simulink model "w3_warplab_buffers"  (Simulink 7.7)
settings: Solver=VariableStepDiscrete  SolverMode=SingleTasking  StartTime=0.0  StopTime=200000  RelTol=1e-3
InitFcn:
  | w3_warplab_buffers_init
StartFcn:
  | w3_warplab_buffers_init
values from neighbouring files (symbols this model uses):
  NumSamps_Rx_IQ = 2^15    (= 32768)    [w3_warplab_buffers_init.m]
  NumSamps_Rx_RSSI = 2^13    (= 8192)    [w3_warplab_buffers_init.m]
  NumSamps_Tx_IQ = 2^15    (= 32768)    [w3_warplab_buffers_init.m]
undefined symbols (not defined in the file or in its folder): gcbh, xlBlockLoadCallback, xlGetNormalizedPeriod
libraries: xbsIndex_r4 x1266, xbsEDKLib_r4 x1
(part 6 of 9)

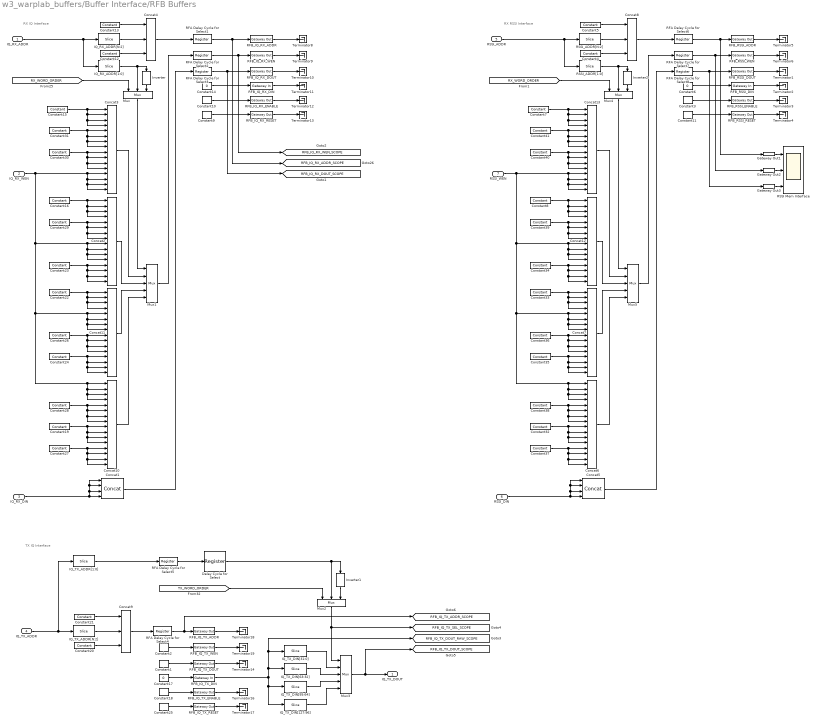
== system w3_warplab_buffers/Buffer Interface/RFB Buffers ==
  note: RX IQ Interface
  note: TX IQ Interface
  note: RX RSSI Interface
  IQ_RX_ADDR : Inport
  IQ_RX_WEN : Inport  Port=2
  IQ_RX_DIN : Inport  Port=3
  IQ_TX_ADDR : Inport  Port=4
  RSSI_ADDR : Inport  Port=5
  RSSI_DIN : Inport  Port=6
  RSSI_WEN : Inport  Port=7
  Concat1 : xbsIndex_r4/Concat  num_inputs=4  dbl_ovrd=off  block_type=concat
  Concat{2..3,6..7,10..13} (8 alike) : xbsIndex_r4/Concat  num_inputs=16  dbl_ovrd=off  block_type=concat
  Concat4 : xbsIndex_r4/Concat  num_inputs=3  dbl_ovrd=off  block_type=concat
  Concat5 : xbsIndex_r4/Concat  num_inputs=4  dbl_ovrd=off  block_type=concat
  Concat8 : xbsIndex_r4/Concat  num_inputs=3  dbl_ovrd=off  block_type=concat
  Concat9 : xbsIndex_r4/Concat  num_inputs=3  dbl_ovrd=off  block_type=concat
  Constant1 : xbsIndex_r4/Constant  const=0  gui_display_data_type=Fixed-point  arith_type=Unsigned  n_bits=128  bin_pt=0  preci_type=Single  exp_width=8  frac_width=24  explicit_period=off  period=1  equ=P=C  opselect=C  inp2=PCIN>>17  opr=+  inp1=P  carry=CIN  dbl_ovrd=off  block_type=constant
      settings: block_version=10.1.2
  Constant10 : xbsIndex_r4/Constant  const=1  gui_display_data_type=Boolean  arith_type=Boolean  n_bits=32  bin_pt=0  preci_type=Single  exp_width=8  frac_width=24  explicit_period=off  period=1  equ=P=C  opselect=C  inp2=PCIN>>17  opr=+  inp1=P  carry=CIN  dbl_ovrd=off  block_type=constant
      settings: block_version=10.1.2
  Constant11 : xbsIndex_r4/Constant  const=0  gui_display_data_type=Boolean  arith_type=Boolean  n_bits=32  bin_pt=0  preci_type=Single  exp_width=8  frac_width=24  explicit_period=off  period=1  equ=P=C  opselect=C  inp2=PCIN>>17  opr=+  inp1=P  carry=CIN  dbl_ovrd=off  block_type=constant
      settings: block_version=10.1.2
  Constant12 : xbsIndex_r4/Constant  const=0  gui_display_data_type=Fixed-point  arith_type=Unsigned  n_bits=4  bin_pt=0  preci_type=Single  exp_width=8  frac_width=24  explicit_period=off  period=1  equ=P=C  opselect=C  inp2=PCIN>>17  opr=+  inp1=P  carry=CIN  dbl_ovrd=off  block_type=constant
  Constant13 : xbsIndex_r4/Constant  const=0  gui_display_data_type=Fixed-point  arith_type=Unsigned  n_bits=30 - ceil(log2(NumSamps_Rx_IQ))  bin_pt=0  preci_type=Single  exp_width=8  frac_width=24  explicit_period=off  period=1  equ=P=C  opselect=C  inp2=PCIN>>17  opr=+  inp1=P  carry=CIN  dbl_ovrd=off  block_type=constant
  Constant14 : Constant  Value=0
  Constant{7..8,15..16,19,22..24,26..41} (24 alike) : xbsIndex_r4/Constant  const=0  gui_display_data_type=Boolean  arith_type=Boolean  n_bits=1  bin_pt=0  preci_type=Single  exp_width=8  frac_width=24  explicit_period=off  period=1  equ=P=C  opselect=C  inp2=PCIN>>17  opr=+  inp1=P  carry=CIN  dbl_ovrd=off  block_type=constant
  Constant17 : Constant  Value=0
  Constant18 : xbsIndex_r4/Constant  const=1  gui_display_data_type=Boolean  arith_type=Boolean  n_bits=32  bin_pt=0  preci_type=Single  exp_width=8  frac_width=24  explicit_period=off  period=1  equ=P=C  opselect=C  inp2=PCIN>>17  opr=+  inp1=P  carry=CIN  dbl_ovrd=off  block_type=constant
      settings: block_version=10.1.2
  Constant2 : xbsIndex_r4/Constant  const=0  gui_display_data_type=Fixed-point  arith_type=Unsigned  n_bits=16  bin_pt=0  preci_type=Single  exp_width=8  frac_width=24  explicit_period=off  period=1  equ=P=C  opselect=C  inp2=PCIN>>17  opr=+  inp1=P  carry=CIN  dbl_ovrd=off  block_type=constant
      settings: block_version=10.1.2
  Constant20 : xbsIndex_r4/Constant  const=0  gui_display_data_type=Fixed-point  arith_type=Unsigned  n_bits=4  bin_pt=0  preci_type=Single  exp_width=8  frac_width=24  explicit_period=off  period=1  equ=P=C  opselect=C  inp2=PCIN>>17  opr=+  inp1=P  carry=CIN  dbl_ovrd=off  block_type=constant
  Constant21 : xbsIndex_r4/Constant  const=0  gui_display_data_type=Fixed-point  arith_type=Unsigned  n_bits=30 - ceil(log2(NumSamps_Tx_IQ))  bin_pt=0  preci_type=Single  exp_width=8  frac_width=24  explicit_period=off  period=1  equ=P=C  opselect=C  inp2=PCIN>>17  opr=+  inp1=P  carry=CIN  dbl_ovrd=off  block_type=constant
  Constant25 : xbsIndex_r4/Constant  const=0  gui_display_data_type=Boolean  arith_type=Boolean  n_bits=32  bin_pt=0  preci_type=Single  exp_width=8  frac_width=24  explicit_period=off  period=1  equ=P=C  opselect=C  inp2=PCIN>>17  opr=+  inp1=P  carry=CIN  dbl_ovrd=off  block_type=constant
      settings: block_version=10.1.2
  Constant3 : xbsIndex_r4/Constant  const=1  gui_display_data_type=Boolean  arith_type=Boolean  n_bits=32  bin_pt=0  preci_type=Single  exp_width=8  frac_width=24  explicit_period=off  period=1  equ=P=C  opselect=C  inp2=PCIN>>17  opr=+  inp1=P  carry=CIN  dbl_ovrd=off  block_type=constant
      settings: block_version=10.1.2
  Constant4 : xbsIndex_r4/Constant  const=0  gui_display_data_type=Fixed-point  arith_type=Unsigned  n_bits=4  bin_pt=0  preci_type=Single  exp_width=8  frac_width=24  explicit_period=off  period=1  equ=P=C  opselect=C  inp2=PCIN>>17  opr=+  inp1=P  carry=CIN  dbl_ovrd=off  block_type=constant
  Constant5 : xbsIndex_r4/Constant  const=0  gui_display_data_type=Fixed-point  arith_type=Unsigned  n_bits=31 - ceil(log2(NumSamps_Rx_RSSI))  bin_pt=0  preci_type=Single  exp_width=8  frac_width=24  explicit_period=off  period=1  equ=P=C  opselect=C  inp2=PCIN>>17  opr=+  inp1=P  carry=CIN  dbl_ovrd=off  block_type=constant
  Constant6 : Constant  Value=0
  Constant9 : xbsIndex_r4/Constant  const=0  gui_display_data_type=Boolean  arith_type=Boolean  n_bits=32  bin_pt=0  preci_type=Single  exp_width=8  frac_width=24  explicit_period=off  period=1  equ=P=C  opselect=C  inp2=PCIN>>17  opr=+  inp1=P  carry=CIN  dbl_ovrd=off  block_type=constant
      settings: block_version=10.1.2
  Delay Cycle for Select : xbsIndex_r4/Register  init=0  rst=off  en=off  dbl_ovrd=off  block_type=register
  Gateway Out1 : xbsIndex_r4/Gateway Out  inherit_from_input=off  hdl_port=off  timing_constraint=None  locs_specified=off  LOCs={}  UseAsDAC=off  DACChannel='1'  block_type=gatewayout
      settings: infoedit="Gateway out block.  Converts Xilinx fixed point inputs into ouputs of type Simulink integer, double, or fixed point.<P><P>Hardware notes:  In hardware these blocks become top level output ports or are discarded, depending on how they are configured."  block_version=10.1.2
  Gateway Out2 : xbsIndex_r4/Gateway Out  inherit_from_input=off  hdl_port=off  timing_constraint=None  locs_specified=off  LOCs={}  UseAsDAC=off  DACChannel='1'  block_type=gatewayout
      settings: infoedit="Gateway out block.  Converts Xilinx fixed point inputs into ouputs of type Simulink integer, double, or fixed point.<P><P>Hardware notes:  In hardware these blocks become top level output ports or are discarded, depending on how they are configured."  block_version=10.1.2
  Gateway Out3 : xbsIndex_r4/Gateway Out  inherit_from_input=off  hdl_port=off  timing_constraint=None  locs_specified=off  LOCs={}  UseAsDAC=off  DACChannel='1'  block_type=gatewayout
      settings: infoedit="Gateway out block.  Converts Xilinx fixed point inputs into ouputs of type Simulink integer, double, or fixed point.<P><P>Hardware notes:  In hardware these blocks become top level output ports or are discarded, depending on how they are configured."  block_version=10.1.2
  IQ_RX_ADDR[1:0] : xbsIndex_r4/Slice  nbits=2  boolean_output=off  mode=Lower Bit Location + Width  bit1=0  base1=MSB of Input  bit0=0  base0=LSB of Input  dbl_ovrd=off  block_type=slice
  IQ_RX_ADDR[N:2] : xbsIndex_r4/Slice  nbits=ceil(log2(NumSamps_Rx_IQ)) - 2  boolean_output=off  mode=Lower Bit Location + Width  bit1=0  base1=MSB of Input  bit0=2  base0=LSB of Input  dbl_ovrd=off  block_type=slice
  IQ_TX_ADDR[1:0] : xbsIndex_r4/Slice  nbits=2  boolean_output=off  mode=Lower Bit Location + Width  bit1=0  base1=MSB of Input  bit0=0  base0=LSB of Input  dbl_ovrd=off  block_type=slice
  IQ_TX_ADDR[N:2] : xbsIndex_r4/Slice  nbits=ceil(log2(NumSamps_Tx_IQ)) - 2  boolean_output=off  mode=Lower Bit Location + Width  bit1=0  base1=MSB of Input  bit0=2  base0=LSB of Input  dbl_ovrd=off  block_type=slice
  IQ_TX_DIN[127:96] : xbsIndex_r4/Slice  nbits=32  boolean_output=off  mode=Lower Bit Location + Width  bit1=0  base1=MSB of Input  bit0=96  base0=LSB of Input  dbl_ovrd=off  block_type=slice
  IQ_TX_DIN[31:0] : xbsIndex_r4/Slice  nbits=32  boolean_output=off  mode=Lower Bit Location + Width  bit1=0  base1=MSB of Input  bit0=0  base0=LSB of Input  dbl_ovrd=off  block_type=slice
  IQ_TX_DIN[63:32] : xbsIndex_r4/Slice  nbits=32  boolean_output=off  mode=Lower Bit Location + Width  bit1=0  base1=MSB of Input  bit0=32  base0=LSB of Input  dbl_ovrd=off  block_type=slice
  IQ_TX_DIN[95:64] : xbsIndex_r4/Slice  nbits=32  boolean_output=off  mode=Lower Bit Location + Width  bit1=0  base1=MSB of Input  bit0=64  base0=LSB of Input  dbl_ovrd=off  block_type=slice
  Inverter : xbsIndex_r4/Inverter  en=off  latency=0  dbl_ovrd=off  block_type=inv
  Inverter1 : xbsIndex_r4/Inverter  en=off  latency=0  dbl_ovrd=off  block_type=inv
  Inverter2 : xbsIndex_r4/Inverter  en=off  latency=0  dbl_ovrd=off  block_type=inv
  Mux : xbsIndex_r4/Mux  inputs=2  en=off  latency=0  precision=Full  arith_type=Unsigned  n_bits=16  bin_pt=14  quantization=Truncate  overflow=Wrap  dbl_ovrd=off  block_type=mux
  Mux1 : xbsIndex_r4/Mux  inputs=4  en=off  latency=0  precision=Full  arith_type=Unsigned  n_bits=16  bin_pt=14  quantization=Truncate  overflow=Wrap  dbl_ovrd=off  block_type=mux
  Mux2 : xbsIndex_r4/Mux  inputs=2  en=off  latency=0  precision=Full  arith_type=Unsigned  n_bits=16  bin_pt=14  quantization=Truncate  overflow=Wrap  dbl_ovrd=off  block_type=mux
  Mux3 : xbsIndex_r4/Mux  inputs=4  en=off  latency=0  precision=Full  arith_type=Unsigned  n_bits=16  bin_pt=14  quantization=Truncate  overflow=Wrap  dbl_ovrd=off  block_type=mux
  Mux4 : xbsIndex_r4/Mux  inputs=2  en=off  latency=0  precision=Full  arith_type=Unsigned  n_bits=16  bin_pt=14  quantization=Truncate  overflow=Wrap  dbl_ovrd=off  block_type=mux
  Mux5 : xbsIndex_r4/Mux  inputs=4  en=off  latency=0  precision=Full  arith_type=Unsigned  n_bits=16  bin_pt=14  quantization=Truncate  overflow=Wrap  dbl_ovrd=off  block_type=mux
  RFA Delay Cycle for Select{1..8} (8 alike) : xbsIndex_r4/Register  init=0  rst=off  en=off  dbl_ovrd=off  block_type=register
  RFB_IQ_RX_ADDR : xbsIndex_r4/Gateway Out  inherit_from_input=off  hdl_port=on  timing_constraint=None  locs_specified=off  LOCs={}  UseAsDAC=off  DACChannel='1'  block_type=gatewayout
  RFB_IQ_RX_DIN : xbsIndex_r4/Gateway In  gui_display_data_type=Fixed-point  arith_type=Unsigned  n_bits=128  bin_pt=0  preci_type=Single  exp_width=8  frac_width=24  quantization="Round  (unbiased: +/- Inf)"  overflow=Saturate  period=1  dbl_ovrd=off  timing_constraint=None  locs_specified=off  LOCs={}  UseAsADC=off  ADCChannel='1'  inherit_from_input=off  hdl_port=on  block_type=gatewayin
  RFB_IQ_RX_DOUT : xbsIndex_r4/Gateway Out  inherit_from_input=off  hdl_port=on  timing_constraint=None  locs_specified=off  LOCs={}  UseAsDAC=off  DACChannel='1'  block_type=gatewayout
  RFB_IQ_RX_ENABLE : xbsIndex_r4/Gateway Out  inherit_from_input=off  hdl_port=on  timing_constraint=None  locs_specified=off  LOCs={}  UseAsDAC=off  DACChannel='1'  block_type=gatewayout
  RFB_IQ_RX_RESET : xbsIndex_r4/Gateway Out  inherit_from_input=off  hdl_port=on  timing_constraint=None  locs_specified=off  LOCs={}  UseAsDAC=off  DACChannel='1'  block_type=gatewayout
  RFB_IQ_RX_WEN : xbsIndex_r4/Gateway Out  inherit_from_input=off  hdl_port=on  timing_constraint=None  locs_specified=off  LOCs={}  UseAsDAC=off  DACChannel='1'  block_type=gatewayout
  RFB_IQ_TX_ADDR : xbsIndex_r4/Gateway Out  inherit_from_input=off  hdl_port=on  timing_constraint=None  locs_specified=off  LOCs={}  UseAsDAC=off  DACChannel='1'  block_type=gatewayout
  RFB_IQ_TX_DIN : xbsIndex_r4/Gateway In  gui_display_data_type=Fixed-point  arith_type=Unsigned  n_bits=128  bin_pt=0  preci_type=Single  exp_width=8  frac_width=24  quantization="Round  (unbiased: +/- Inf)"  overflow=Saturate  period=1  dbl_ovrd=off  timing_constraint=None  locs_specified=off  LOCs={}  UseAsADC=off  ADCChannel='1'  inherit_from_input=off  hdl_port=on  block_type=gatewayin
  RFB_IQ_TX_DOUT : xbsIndex_r4/Gateway Out  inherit_from_input=off  hdl_port=on  timing_constraint=None  locs_specified=off  LOCs={}  UseAsDAC=off  DACChannel='1'  block_type=gatewayout
  RFB_IQ_TX_ENABLE : xbsIndex_r4/Gateway Out  inherit_from_input=off  hdl_port=on  timing_constraint=None  locs_specified=off  LOCs={}  UseAsDAC=off  DACChannel='1'  block_type=gatewayout
  RFB_IQ_TX_RESET : xbsIndex_r4/Gateway Out  inherit_from_input=off  hdl_port=on  timing_constraint=None  locs_specified=off  LOCs={}  UseAsDAC=off  DACChannel='1'  block_type=gatewayout
  RFB_IQ_TX_WEN : xbsIndex_r4/Gateway Out  inherit_from_input=off  hdl_port=on  timing_constraint=None  locs_specified=off  LOCs={}  UseAsDAC=off  DACChannel='1'  block_type=gatewayout
  RFB_RSSI_ADDR : xbsIndex_r4/Gateway Out  inherit_from_input=off  hdl_port=on  timing_constraint=None  locs_specified=off  LOCs={}  UseAsDAC=off  DACChannel='1'  block_type=gatewayout
  RFB_RSSI_DIN : xbsIndex_r4/Gateway In  gui_display_data_type=Fixed-point  arith_type=Unsigned  n_bits=128  bin_pt=0  preci_type=Single  exp_width=8  frac_width=24  quantization="Round  (unbiased: +/- Inf)"  overflow=Saturate  period=1  dbl_ovrd=off  timing_constraint=None  locs_specified=off  LOCs={}  UseAsADC=off  ADCChannel='1'  inherit_from_input=off  hdl_port=on  block_type=gatewayin
  RFB_RSSI_DOUT : xbsIndex_r4/Gateway Out  inherit_from_input=off  hdl_port=on  timing_constraint=None  locs_specified=off  LOCs={}  UseAsDAC=off  DACChannel='1'  block_type=gatewayout
  RFB_RSSI_ENABLE : xbsIndex_r4/Gateway Out  inherit_from_input=off  hdl_port=on  timing_constraint=None  locs_specified=off  LOCs={}  UseAsDAC=off  DACChannel='1'  block_type=gatewayout
  RFB_RSSI_RESET : xbsIndex_r4/Gateway Out  inherit_from_input=off  hdl_port=on  timing_constraint=None  locs_specified=off  LOCs={}  UseAsDAC=off  DACChannel='1'  block_type=gatewayout
  RFB_RSSI_WEN : xbsIndex_r4/Gateway Out  inherit_from_input=off  hdl_port=on  timing_constraint=None  locs_specified=off  LOCs={}  UseAsDAC=off  DACChannel='1'  block_type=gatewayout
  RSSI Mem Interface : Scope  NumInputPorts=3
      settings: TimeRange=70000  YMin=0~0~0  YMax=1~1~1  SaveName=ScopeData6
  RSSI_ADDR[1:0] : xbsIndex_r4/Slice  nbits=2  boolean_output=off  mode=Lower Bit Location + Width  bit1=0  base1=MSB of Input  bit0=0  base0=LSB of Input  dbl_ovrd=off  block_type=slice
  RSSI_ADDR[N:2] : xbsIndex_r4/Slice  nbits=ceil(log2(NumSamps_Rx_RSSI)) - 3  boolean_output=off  mode=Lower Bit Location + Width  bit1=0  base1=MSB of Input  bit0=2  base0=LSB of Input  dbl_ovrd=off  block_type=slice
  Terminator{1..6,8..14,16..19} (17 alike) : Terminator
  IQ_TX_DOUT : Outport
  tag scope: RFB_IQ_RX_ADDR_SCOPE=global, RFB_IQ_RX_DOUT_SCOPE=global, RFB_IQ_RX_WEN_SCOPE=global, RFB_IQ_TX_ADDR_SCOPE=global, RFB_IQ_TX_DOUT_RAW_SCOPE=global, RFB_IQ_TX_DOUT_SCOPE=global, RFB_IQ_TX_SEL_SCOPE=global
  wires:
  IQ_RX_ADDR/1 -> IQ_RX_ADDR[1:0]/1, IQ_RX_ADDR[N:2]/1
  IQ_RX_DIN/1 -> Concat1/4, Concat1/3, Concat1/2, Concat1/1
  RFB_IQ_RX_ADDR/1 -> Terminator8/1
  RFB_IQ_RX_WEN/1 -> Terminator9/1
  RFB_IQ_RX_DOUT/1 -> Terminator10/1
  RFB_IQ_RX_ENABLE/1 -> Terminator12/1
  RFB_IQ_RX_RESET/1 -> Terminator13/1
  RFB_IQ_RX_DIN/1 -> Terminator11/1
  Constant9/1 -> RFB_IQ_RX_RESET/1
  Constant10/1 -> RFB_IQ_RX_ENABLE/1
  Constant14/1 -> RFB_IQ_RX_DIN/1
  Constant13/1 -> Concat4/1
  IQ_RX_ADDR[N:2]/1 -> Concat4/2
  Constant12/1 -> Concat4/3
  Concat4/1 -> RFA Delay Cycle for Select1/1
  Mux1/1 -> RFA Delay Cycle for Select2/1
  IQ_TX_ADDR/1 -> IQ_TX_ADDR[1:0]/1, IQ_TX_ADDR[N:2]/1
  RFB_IQ_TX_ADDR/1 -> Terminator18/1
  RFB_IQ_TX_WEN/1 -> Terminator19/1
  RFB_IQ_TX_DOUT/1 -> Terminator14/1
  RFB_IQ_TX_ENABLE/1 -> Terminator16/1
  RFB_IQ_TX_RESET/1 -> Terminator17/1
  Constant25/1 -> RFB_IQ_TX_RESET/1
  Constant18/1 -> RFB_IQ_TX_ENABLE/1
  Constant21/1 -> Concat9/1
  IQ_TX_ADDR[N:2]/1 -> Concat9/2
  Constant20/1 -> Concat9/3
  Concat9/1 -> RFA Delay Cycle for Select4/1
  Constant2/1 -> RFB_IQ_TX_WEN/1
  Constant1/1 -> RFB_IQ_TX_DOUT/1
  IQ_TX_ADDR[1:0]/1 -> RFA Delay Cycle for Select5/1
  RFB_IQ_TX_DIN/1 -> IQ_TX_DIN[63:32]/1, IQ_TX_DIN[31:0]/1, [RFB_IQ_TX_DOUT_RAW_SCOPE], IQ_TX_DIN[127:96]/1, IQ_TX_DIN[95:64]/1
  IQ_TX_DIN[31:0]/1 -> Mux3/2
  IQ_TX_DIN[63:32]/1 -> Mux3/3
  RFA Delay Cycle for Select1/1 -> RFB_IQ_RX_ADDR/1, [RFB_IQ_RX_ADDR_SCOPE]
  RFA Delay Cycle for Select2/1 -> RFB_IQ_RX_WEN/1, [RFB_IQ_RX_WEN_SCOPE]
  Constant17/1 -> RFB_IQ_TX_DIN/1
  RFA Delay Cycle for Select3/1 -> RFB_IQ_RX_DOUT/1, [RFB_IQ_RX_DOUT_SCOPE]
  Concat1/1 -> RFA Delay Cycle for Select3/1
  RFA Delay Cycle for Select4/1 -> RFB_IQ_TX_ADDR/1, [RFB_IQ_TX_ADDR_SCOPE]
  RFA Delay Cycle for Select5/1 -> Delay Cycle for Select/1
  IQ_RX_ADDR[1:0]/1 -> Inverter/1, Mux/2
  Inverter/1 -> Mux/3
  Mux/1 -> Mux1/1
  Inverter1/1 -> Mux2/3
  Delay Cycle for Select/1 -> Inverter1/1, Mux2/2
  Mux2/1 -> Mux3/1, [RFB_IQ_TX_SEL_SCOPE]
  [RX_WORD_ORDER] -> Mux/1
  Mux3/1 -> IQ_TX_DOUT/1, [RFB_IQ_TX_DOUT_SCOPE]
  RSSI_ADDR/1 -> RSSI_ADDR[1:0]/1, RSSI_ADDR[N:2]/1
  RFB_RSSI_ADDR/1 -> Terminator5/1
  RFB_RSSI_WEN/1 -> Terminator6/1
  RFB_RSSI_DOUT/1 -> Terminator1/1
  RFB_RSSI_ENABLE/1 -> Terminator3/1
  RFB_RSSI_RESET/1 -> Terminator4/1
  RFB_RSSI_DIN/1 -> Terminator2/1
  Constant11/1 -> RFB_RSSI_RESET/1
  Constant3/1 -> RFB_RSSI_ENABLE/1
  Constant6/1 -> RFB_RSSI_DIN/1
  Constant5/1 -> Concat8/1
  RSSI_ADDR[N:2]/1 -> Concat8/2
  Constant4/1 -> Concat8/3
  Concat8/1 -> RFA Delay Cycle for Select6/1
  RFA Delay Cycle for Select6/1 -> RFB_RSSI_ADDR/1, Gateway Out1/1
  RFA Delay Cycle for Select7/1 -> RFB_RSSI_WEN/1, Gateway Out2/1
  RFA Delay Cycle for Select8/1 -> RFB_RSSI_DOUT/1, Gateway Out3/1
  RSSI_ADDR[1:0]/1 -> Inverter2/1, Mux4/2
  Inverter2/1 -> Mux4/3
  Gateway Out1/1 -> RSSI Mem Interface/1
  Gateway Out2/1 -> RSSI Mem Interface/2
  Gateway Out3/1 -> RSSI Mem Interface/3
  Constant15/1 -> Concat3/1, Concat3/2, Concat3/3, Concat3/4
  IQ_RX_WEN/1 -> Concat3/13, Concat3/14, Concat3/15, Concat3/16, Concat2/9, Concat2/10, Concat2/11, Concat2/12, Concat11/5, Concat11/6, Concat11/7, Concat11/8, Concat10/1, Concat10/2, Concat10/3, Concat10/4
  Constant16/1 -> Concat2/1, Concat2/2, Concat2/3, Concat2/4
  Constant23/1 -> Concat2/13, Concat2/14, Concat2/15, Concat2/16
  Constant22/1 -> Concat11/3, Concat11/4, Concat11/2, Concat11/1
  Constant24/1 -> Concat11/15, Concat11/16, Concat11/14, Concat11/13
  Constant26/1 -> Concat11/11, Concat11/12, Concat11/10, Concat11/9
  Constant27/1 -> Concat10/15, Concat10/16, Concat10/14, Concat10/13
  Constant19/1 -> Concat10/11, Concat10/12, Concat10/10, Concat10/9
  Constant28/1 -> Concat10/7, Concat10/8, Concat10/6, Concat10/5
  Constant29/1 -> Concat2/7, Concat2/8, Concat2/6, Concat2/5
  Constant30/1 -> Concat3/11, Concat3/12, Concat3/10, Concat3/9
  Constant31/1 -> Concat3/7, Concat3/8, Concat3/6, Concat3/5
  Concat3/1 -> Mux1/2
  Concat2/1 -> Mux1/3
  Concat11/1 -> Mux1/4
  Concat10/1 -> Mux1/5
  [RX_WORD_ORDER] -> Mux4/1
  [TX_WORD_ORDER] -> Mux2/1
  RSSI_DIN/1 -> Concat5/4, Concat5/3, Concat5/2, Concat5/1
  Mux5/1 -> RFA Delay Cycle for Select7/1
  Concat5/1 -> RFA Delay Cycle for Select8/1
  Mux4/1 -> Mux5/1
  Constant7/1 -> Concat13/1, Concat13/2, Concat13/3, Concat13/4
  RSSI_WEN/1 -> Concat13/13, Concat13/14, Concat13/15, Concat13/16, Concat12/9, Concat12/10, Concat12/11, Concat12/12, Concat7/5, Concat7/6, Concat7/7, Concat7/8, Concat6/1, Concat6/2, Concat6/3, Concat6/4
  Constant8/1 -> Concat12/1, Concat12/2, Concat12/3, Concat12/4
  Constant34/1 -> Concat12/13, Concat12/14, Concat12/15, Concat12/16
  Constant33/1 -> Concat7/3, Concat7/4, Concat7/2, Concat7/1
  Constant35/1 -> Concat7/15, Concat7/16, Concat7/14, Concat7/13
  Constant36/1 -> Concat7/11, Concat7/12, Concat7/10, Concat7/9
  Constant37/1 -> Concat6/15, Concat6/16, Concat6/14, Concat6/13
  Constant32/1 -> Concat6/11, Concat6/12, Concat6/10, Concat6/9
  Constant38/1 -> Concat6/7, Concat6/8, Concat6/6, Concat6/5
  Constant39/1 -> Concat12/7, Concat12/8, Concat12/6, Concat12/5
  Constant40/1 -> Concat13/11, Concat13/12, Concat13/10, Concat13/9
  Constant41/1 -> Concat13/7, Concat13/8, Concat13/6, Concat13/5
  Concat13/1 -> Mux5/2
  Concat12/1 -> Mux5/3
  Concat7/1 -> Mux5/4
  Concat6/1 -> Mux5/5
  IQ_TX_DIN[95:64]/1 -> Mux3/4
  IQ_TX_DIN[127:96]/1 -> Mux3/5

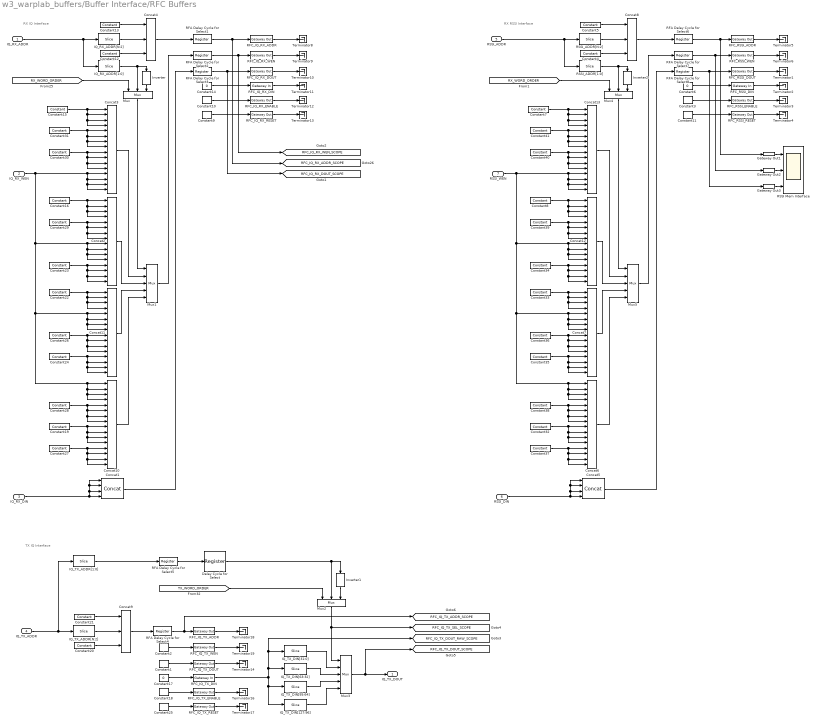
== system w3_warplab_buffers/Buffer Interface/RFC Buffers ==
  note: RX IQ Interface
  note: TX IQ Interface
  note: RX RSSI Interface
  IQ_RX_ADDR : Inport
  IQ_RX_WEN : Inport  Port=2
  IQ_RX_DIN : Inport  Port=3
  IQ_TX_ADDR : Inport  Port=4
  RSSI_ADDR : Inport  Port=5
  RSSI_DIN : Inport  Port=6
  RSSI_WEN : Inport  Port=7
  Concat1 : xbsIndex_r4/Concat  num_inputs=4  dbl_ovrd=off  block_type=concat
  Concat{2..3,6..7,10..13} (8 alike) : xbsIndex_r4/Concat  num_inputs=16  dbl_ovrd=off  block_type=concat
  Concat4 : xbsIndex_r4/Concat  num_inputs=3  dbl_ovrd=off  block_type=concat
  Concat5 : xbsIndex_r4/Concat  num_inputs=4  dbl_ovrd=off  block_type=concat
  Concat8 : xbsIndex_r4/Concat  num_inputs=3  dbl_ovrd=off  block_type=concat
  Concat9 : xbsIndex_r4/Concat  num_inputs=3  dbl_ovrd=off  block_type=concat
  Constant1 : xbsIndex_r4/Constant  const=0  gui_display_data_type=Fixed-point  arith_type=Unsigned  n_bits=128  bin_pt=0  preci_type=Single  exp_width=8  frac_width=24  explicit_period=off  period=1  equ=P=C  opselect=C  inp2=PCIN>>17  opr=+  inp1=P  carry=CIN  dbl_ovrd=off  block_type=constant
      settings: block_version=10.1.2
  Constant10 : xbsIndex_r4/Constant  const=1  gui_display_data_type=Boolean  arith_type=Boolean  n_bits=32  bin_pt=0  preci_type=Single  exp_width=8  frac_width=24  explicit_period=off  period=1  equ=P=C  opselect=C  inp2=PCIN>>17  opr=+  inp1=P  carry=CIN  dbl_ovrd=off  block_type=constant
      settings: block_version=10.1.2
  Constant11 : xbsIndex_r4/Constant  const=0  gui_display_data_type=Boolean  arith_type=Boolean  n_bits=32  bin_pt=0  preci_type=Single  exp_width=8  frac_width=24  explicit_period=off  period=1  equ=P=C  opselect=C  inp2=PCIN>>17  opr=+  inp1=P  carry=CIN  dbl_ovrd=off  block_type=constant
      settings: block_version=10.1.2
  Constant12 : xbsIndex_r4/Constant  const=0  gui_display_data_type=Fixed-point  arith_type=Unsigned  n_bits=4  bin_pt=0  preci_type=Single  exp_width=8  frac_width=24  explicit_period=off  period=1  equ=P=C  opselect=C  inp2=PCIN>>17  opr=+  inp1=P  carry=CIN  dbl_ovrd=off  block_type=constant
  Constant13 : xbsIndex_r4/Constant  const=0  gui_display_data_type=Fixed-point  arith_type=Unsigned  n_bits=30 - ceil(log2(NumSamps_Rx_IQ))  bin_pt=0  preci_type=Single  exp_width=8  frac_width=24  explicit_period=off  period=1  equ=P=C  opselect=C  inp2=PCIN>>17  opr=+  inp1=P  carry=CIN  dbl_ovrd=off  block_type=constant
  Constant14 : Constant  Value=0
  Constant{7..8,15..16,19,22..24,26..41} (24 alike) : xbsIndex_r4/Constant  const=0  gui_display_data_type=Boolean  arith_type=Boolean  n_bits=1  bin_pt=0  preci_type=Single  exp_width=8  frac_width=24  explicit_period=off  period=1  equ=P=C  opselect=C  inp2=PCIN>>17  opr=+  inp1=P  carry=CIN  dbl_ovrd=off  block_type=constant
  Constant17 : Constant  Value=0
  Constant18 : xbsIndex_r4/Constant  const=1  gui_display_data_type=Boolean  arith_type=Boolean  n_bits=32  bin_pt=0  preci_type=Single  exp_width=8  frac_width=24  explicit_period=off  period=1  equ=P=C  opselect=C  inp2=PCIN>>17  opr=+  inp1=P  carry=CIN  dbl_ovrd=off  block_type=constant
      settings: block_version=10.1.2
  Constant2 : xbsIndex_r4/Constant  const=0  gui_display_data_type=Fixed-point  arith_type=Unsigned  n_bits=16  bin_pt=0  preci_type=Single  exp_width=8  frac_width=24  explicit_period=off  period=1  equ=P=C  opselect=C  inp2=PCIN>>17  opr=+  inp1=P  carry=CIN  dbl_ovrd=off  block_type=constant
      settings: block_version=10.1.2
  Constant20 : xbsIndex_r4/Constant  const=0  gui_display_data_type=Fixed-point  arith_type=Unsigned  n_bits=4  bin_pt=0  preci_type=Single  exp_width=8  frac_width=24  explicit_period=off  period=1  equ=P=C  opselect=C  inp2=PCIN>>17  opr=+  inp1=P  carry=CIN  dbl_ovrd=off  block_type=constant
  Constant21 : xbsIndex_r4/Constant  const=0  gui_display_data_type=Fixed-point  arith_type=Unsigned  n_bits=30 - ceil(log2(NumSamps_Tx_IQ))  bin_pt=0  preci_type=Single  exp_width=8  frac_width=24  explicit_period=off  period=1  equ=P=C  opselect=C  inp2=PCIN>>17  opr=+  inp1=P  carry=CIN  dbl_ovrd=off  block_type=constant
  Constant25 : xbsIndex_r4/Constant  const=0  gui_display_data_type=Boolean  arith_type=Boolean  n_bits=32  bin_pt=0  preci_type=Single  exp_width=8  frac_width=24  explicit_period=off  period=1  equ=P=C  opselect=C  inp2=PCIN>>17  opr=+  inp1=P  carry=CIN  dbl_ovrd=off  block_type=constant
      settings: block_version=10.1.2
  Constant3 : xbsIndex_r4/Constant  const=1  gui_display_data_type=Boolean  arith_type=Boolean  n_bits=32  bin_pt=0  preci_type=Single  exp_width=8  frac_width=24  explicit_period=off  period=1  equ=P=C  opselect=C  inp2=PCIN>>17  opr=+  inp1=P  carry=CIN  dbl_ovrd=off  block_type=constant
      settings: block_version=10.1.2
  Constant4 : xbsIndex_r4/Constant  const=0  gui_display_data_type=Fixed-point  arith_type=Unsigned  n_bits=4  bin_pt=0  preci_type=Single  exp_width=8  frac_width=24  explicit_period=off  period=1  equ=P=C  opselect=C  inp2=PCIN>>17  opr=+  inp1=P  carry=CIN  dbl_ovrd=off  block_type=constant
  Constant5 : xbsIndex_r4/Constant  const=0  gui_display_data_type=Fixed-point  arith_type=Unsigned  n_bits=31 - ceil(log2(NumSamps_Rx_RSSI))  bin_pt=0  preci_type=Single  exp_width=8  frac_width=24  explicit_period=off  period=1  equ=P=C  opselect=C  inp2=PCIN>>17  opr=+  inp1=P  carry=CIN  dbl_ovrd=off  block_type=constant
  Constant6 : Constant  Value=0
  Constant9 : xbsIndex_r4/Constant  const=0  gui_display_data_type=Boolean  arith_type=Boolean  n_bits=32  bin_pt=0  preci_type=Single  exp_width=8  frac_width=24  explicit_period=off  period=1  equ=P=C  opselect=C  inp2=PCIN>>17  opr=+  inp1=P  carry=CIN  dbl_ovrd=off  block_type=constant
      settings: block_version=10.1.2
  Delay Cycle for Select : xbsIndex_r4/Register  init=0  rst=off  en=off  dbl_ovrd=off  block_type=register
  Gateway Out1 : xbsIndex_r4/Gateway Out  inherit_from_input=off  hdl_port=off  timing_constraint=None  locs_specified=off  LOCs={}  UseAsDAC=off  DACChannel='1'  block_type=gatewayout
      settings: infoedit="Gateway out block.  Converts Xilinx fixed point inputs into ouputs of type Simulink integer, double, or fixed point.<P><P>Hardware notes:  In hardware these blocks become top level output ports or are discarded, depending on how they are configured."  block_version=10.1.2
  Gateway Out2 : xbsIndex_r4/Gateway Out  inherit_from_input=off  hdl_port=off  timing_constraint=None  locs_specified=off  LOCs={}  UseAsDAC=off  DACChannel='1'  block_type=gatewayout
      settings: infoedit="Gateway out block.  Converts Xilinx fixed point inputs into ouputs of type Simulink integer, double, or fixed point.<P><P>Hardware notes:  In hardware these blocks become top level output ports or are discarded, depending on how they are configured."  block_version=10.1.2
  Gateway Out3 : xbsIndex_r4/Gateway Out  inherit_from_input=off  hdl_port=off  timing_constraint=None  locs_specified=off  LOCs={}  UseAsDAC=off  DACChannel='1'  block_type=gatewayout
      settings: infoedit="Gateway out block.  Converts Xilinx fixed point inputs into ouputs of type Simulink integer, double, or fixed point.<P><P>Hardware notes:  In hardware these blocks become top level output ports or are discarded, depending on how they are configured."  block_version=10.1.2
  IQ_RX_ADDR[1:0] : xbsIndex_r4/Slice  nbits=2  boolean_output=off  mode=Lower Bit Location + Width  bit1=0  base1=MSB of Input  bit0=0  base0=LSB of Input  dbl_ovrd=off  block_type=slice
  IQ_RX_ADDR[N:2] : xbsIndex_r4/Slice  nbits=ceil(log2(NumSamps_Rx_IQ)) - 2  boolean_output=off  mode=Lower Bit Location + Width  bit1=0  base1=MSB of Input  bit0=2  base0=LSB of Input  dbl_ovrd=off  block_type=slice
  IQ_TX_ADDR[1:0] : xbsIndex_r4/Slice  nbits=2  boolean_output=off  mode=Lower Bit Location + Width  bit1=0  base1=MSB of Input  bit0=0  base0=LSB of Input  dbl_ovrd=off  block_type=slice
  IQ_TX_ADDR[N:2] : xbsIndex_r4/Slice  nbits=ceil(log2(NumSamps_Tx_IQ)) - 2  boolean_output=off  mode=Lower Bit Location + Width  bit1=0  base1=MSB of Input  bit0=2  base0=LSB of Input  dbl_ovrd=off  block_type=slice
  IQ_TX_DIN[127:96] : xbsIndex_r4/Slice  nbits=32  boolean_output=off  mode=Lower Bit Location + Width  bit1=0  base1=MSB of Input  bit0=96  base0=LSB of Input  dbl_ovrd=off  block_type=slice
  IQ_TX_DIN[31:0] : xbsIndex_r4/Slice  nbits=32  boolean_output=off  mode=Lower Bit Location + Width  bit1=0  base1=MSB of Input  bit0=0  base0=LSB of Input  dbl_ovrd=off  block_type=slice
  IQ_TX_DIN[63:32] : xbsIndex_r4/Slice  nbits=32  boolean_output=off  mode=Lower Bit Location + Width  bit1=0  base1=MSB of Input  bit0=32  base0=LSB of Input  dbl_ovrd=off  block_type=slice
  IQ_TX_DIN[95:64] : xbsIndex_r4/Slice  nbits=32  boolean_output=off  mode=Lower Bit Location + Width  bit1=0  base1=MSB of Input  bit0=64  base0=LSB of Input  dbl_ovrd=off  block_type=slice
  Inverter : xbsIndex_r4/Inverter  en=off  latency=0  dbl_ovrd=off  block_type=inv
  Inverter1 : xbsIndex_r4/Inverter  en=off  latency=0  dbl_ovrd=off  block_type=inv
  Inverter2 : xbsIndex_r4/Inverter  en=off  latency=0  dbl_ovrd=off  block_type=inv
  Mux : xbsIndex_r4/Mux  inputs=2  en=off  latency=0  precision=Full  arith_type=Unsigned  n_bits=16  bin_pt=14  quantization=Truncate  overflow=Wrap  dbl_ovrd=off  block_type=mux
  Mux1 : xbsIndex_r4/Mux  inputs=4  en=off  latency=0  precision=Full  arith_type=Unsigned  n_bits=16  bin_pt=14  quantization=Truncate  overflow=Wrap  dbl_ovrd=off  block_type=mux
  Mux2 : xbsIndex_r4/Mux  inputs=2  en=off  latency=0  precision=Full  arith_type=Unsigned  n_bits=16  bin_pt=14  quantization=Truncate  overflow=Wrap  dbl_ovrd=off  block_type=mux
  Mux3 : xbsIndex_r4/Mux  inputs=4  en=off  latency=0  precision=Full  arith_type=Unsigned  n_bits=16  bin_pt=14  quantization=Truncate  overflow=Wrap  dbl_ovrd=off  block_type=mux
  Mux4 : xbsIndex_r4/Mux  inputs=2  en=off  latency=0  precision=Full  arith_type=Unsigned  n_bits=16  bin_pt=14  quantization=Truncate  overflow=Wrap  dbl_ovrd=off  block_type=mux
  Mux5 : xbsIndex_r4/Mux  inputs=4  en=off  latency=0  precision=Full  arith_type=Unsigned  n_bits=16  bin_pt=14  quantization=Truncate  overflow=Wrap  dbl_ovrd=off  block_type=mux
  RFA Delay Cycle for Select{1..8} (8 alike) : xbsIndex_r4/Register  init=0  rst=off  en=off  dbl_ovrd=off  block_type=register
  RFC_IQ_RX_ADDR : xbsIndex_r4/Gateway Out  inherit_from_input=off  hdl_port=on  timing_constraint=None  locs_specified=off  LOCs={}  UseAsDAC=off  DACChannel='1'  block_type=gatewayout
  RFC_IQ_RX_DIN : xbsIndex_r4/Gateway In  gui_display_data_type=Fixed-point  arith_type=Unsigned  n_bits=128  bin_pt=0  preci_type=Single  exp_width=8  frac_width=24  quantization="Round  (unbiased: +/- Inf)"  overflow=Saturate  period=1  dbl_ovrd=off  timing_constraint=None  locs_specified=off  LOCs={}  UseAsADC=off  ADCChannel='1'  inherit_from_input=off  hdl_port=on  block_type=gatewayin
  RFC_IQ_RX_DOUT : xbsIndex_r4/Gateway Out  inherit_from_input=off  hdl_port=on  timing_constraint=None  locs_specified=off  LOCs={}  UseAsDAC=off  DACChannel='1'  block_type=gatewayout
  RFC_IQ_RX_ENABLE : xbsIndex_r4/Gateway Out  inherit_from_input=off  hdl_port=on  timing_constraint=None  locs_specified=off  LOCs={}  UseAsDAC=off  DACChannel='1'  block_type=gatewayout
  RFC_IQ_RX_RESET : xbsIndex_r4/Gateway Out  inherit_from_input=off  hdl_port=on  timing_constraint=None  locs_specified=off  LOCs={}  UseAsDAC=off  DACChannel='1'  block_type=gatewayout
  RFC_IQ_RX_WEN : xbsIndex_r4/Gateway Out  inherit_from_input=off  hdl_port=on  timing_constraint=None  locs_specified=off  LOCs={}  UseAsDAC=off  DACChannel='1'  block_type=gatewayout
  RFC_IQ_TX_ADDR : xbsIndex_r4/Gateway Out  inherit_from_input=off  hdl_port=on  timing_constraint=None  locs_specified=off  LOCs={}  UseAsDAC=off  DACChannel='1'  block_type=gatewayout
  RFC_IQ_TX_DIN : xbsIndex_r4/Gateway In  gui_display_data_type=Fixed-point  arith_type=Unsigned  n_bits=128  bin_pt=0  preci_type=Single  exp_width=8  frac_width=24  quantization="Round  (unbiased: +/- Inf)"  overflow=Saturate  period=1  dbl_ovrd=off  timing_constraint=None  locs_specified=off  LOCs={}  UseAsADC=off  ADCChannel='1'  inherit_from_input=off  hdl_port=on  block_type=gatewayin
  RFC_IQ_TX_DOUT : xbsIndex_r4/Gateway Out  inherit_from_input=off  hdl_port=on  timing_constraint=None  locs_specified=off  LOCs={}  UseAsDAC=off  DACChannel='1'  block_type=gatewayout
  RFC_IQ_TX_ENABLE : xbsIndex_r4/Gateway Out  inherit_from_input=off  hdl_port=on  timing_constraint=None  locs_specified=off  LOCs={}  UseAsDAC=off  DACChannel='1'  block_type=gatewayout
  RFC_IQ_TX_RESET : xbsIndex_r4/Gateway Out  inherit_from_input=off  hdl_port=on  timing_constraint=None  locs_specified=off  LOCs={}  UseAsDAC=off  DACChannel='1'  block_type=gatewayout
  RFC_IQ_TX_WEN : xbsIndex_r4/Gateway Out  inherit_from_input=off  hdl_port=on  timing_constraint=None  locs_specified=off  LOCs={}  UseAsDAC=off  DACChannel='1'  block_type=gatewayout
  RFC_RSSI_ADDR : xbsIndex_r4/Gateway Out  inherit_from_input=off  hdl_port=on  timing_constraint=None  locs_specified=off  LOCs={}  UseAsDAC=off  DACChannel='1'  block_type=gatewayout
  RFC_RSSI_DIN : xbsIndex_r4/Gateway In  gui_display_data_type=Fixed-point  arith_type=Unsigned  n_bits=128  bin_pt=0  preci_type=Single  exp_width=8  frac_width=24  quantization="Round  (unbiased: +/- Inf)"  overflow=Saturate  period=1  dbl_ovrd=off  timing_constraint=None  locs_specified=off  LOCs={}  UseAsADC=off  ADCChannel='1'  inherit_from_input=off  hdl_port=on  block_type=gatewayin
  RFC_RSSI_DOUT : xbsIndex_r4/Gateway Out  inherit_from_input=off  hdl_port=on  timing_constraint=None  locs_specified=off  LOCs={}  UseAsDAC=off  DACChannel='1'  block_type=gatewayout
  RFC_RSSI_ENABLE : xbsIndex_r4/Gateway Out  inherit_from_input=off  hdl_port=on  timing_constraint=None  locs_specified=off  LOCs={}  UseAsDAC=off  DACChannel='1'  block_type=gatewayout
  RFC_RSSI_RESET : xbsIndex_r4/Gateway Out  inherit_from_input=off  hdl_port=on  timing_constraint=None  locs_specified=off  LOCs={}  UseAsDAC=off  DACChannel='1'  block_type=gatewayout
  RFC_RSSI_WEN : xbsIndex_r4/Gateway Out  inherit_from_input=off  hdl_port=on  timing_constraint=None  locs_specified=off  LOCs={}  UseAsDAC=off  DACChannel='1'  block_type=gatewayout
  RSSI Mem Interface : Scope  NumInputPorts=3
      settings: TimeRange=70000  YMin=0~0~0  YMax=1~1~1  SaveName=ScopeData6
  RSSI_ADDR[1:0] : xbsIndex_r4/Slice  nbits=2  boolean_output=off  mode=Lower Bit Location + Width  bit1=0  base1=MSB of Input  bit0=0  base0=LSB of Input  dbl_ovrd=off  block_type=slice
  RSSI_ADDR[N:2] : xbsIndex_r4/Slice  nbits=ceil(log2(NumSamps_Rx_RSSI)) - 3  boolean_output=off  mode=Lower Bit Location + Width  bit1=0  base1=MSB of Input  bit0=2  base0=LSB of Input  dbl_ovrd=off  block_type=slice
  Terminator{1..6,8..14,16..19} (17 alike) : Terminator
  IQ_TX_DOUT : Outport
  tag scope: RFC_IQ_RX_ADDR_SCOPE=global, RFC_IQ_RX_DOUT_SCOPE=global, RFC_IQ_RX_WEN_SCOPE=global, RFC_IQ_TX_ADDR_SCOPE=global, RFC_IQ_TX_DOUT_RAW_SCOPE=global, RFC_IQ_TX_DOUT_SCOPE=global, RFC_IQ_TX_SEL_SCOPE=global
  wires:
  IQ_RX_ADDR/1 -> IQ_RX_ADDR[1:0]/1, IQ_RX_ADDR[N:2]/1
  IQ_RX_DIN/1 -> Concat1/4, Concat1/3, Concat1/2, Concat1/1
  RFC_IQ_RX_ADDR/1 -> Terminator8/1
  RFC_IQ_RX_WEN/1 -> Terminator9/1
  RFC_IQ_RX_DOUT/1 -> Terminator10/1
  RFC_IQ_RX_ENABLE/1 -> Terminator12/1
  RFC_IQ_RX_RESET/1 -> Terminator13/1
  RFC_IQ_RX_DIN/1 -> Terminator11/1
  Constant9/1 -> RFC_IQ_RX_RESET/1
  Constant10/1 -> RFC_IQ_RX_ENABLE/1
  Constant14/1 -> RFC_IQ_RX_DIN/1
  Constant13/1 -> Concat4/1
  IQ_RX_ADDR[N:2]/1 -> Concat4/2
  Constant12/1 -> Concat4/3
  Concat4/1 -> RFA Delay Cycle for Select1/1
  Mux1/1 -> RFA Delay Cycle for Select2/1
  IQ_TX_ADDR/1 -> IQ_TX_ADDR[1:0]/1, IQ_TX_ADDR[N:2]/1
  RFC_IQ_TX_ADDR/1 -> Terminator18/1
  RFC_IQ_TX_WEN/1 -> Terminator19/1
  RFC_IQ_TX_DOUT/1 -> Terminator14/1
  RFC_IQ_TX_ENABLE/1 -> Terminator16/1
  RFC_IQ_TX_RESET/1 -> Terminator17/1
  Constant25/1 -> RFC_IQ_TX_RESET/1
  Constant18/1 -> RFC_IQ_TX_ENABLE/1
  Constant21/1 -> Concat9/1
  IQ_TX_ADDR[N:2]/1 -> Concat9/2
  Constant20/1 -> Concat9/3
  Concat9/1 -> RFA Delay Cycle for Select4/1
  Constant2/1 -> RFC_IQ_TX_WEN/1
  Constant1/1 -> RFC_IQ_TX_DOUT/1
  IQ_TX_ADDR[1:0]/1 -> RFA Delay Cycle for Select5/1
  RFC_IQ_TX_DIN/1 -> IQ_TX_DIN[63:32]/1, IQ_TX_DIN[31:0]/1, [RFC_IQ_TX_DOUT_RAW_SCOPE], IQ_TX_DIN[127:96]/1, IQ_TX_DIN[95:64]/1
  IQ_TX_DIN[31:0]/1 -> Mux3/2
  IQ_TX_DIN[63:32]/1 -> Mux3/3
  RFA Delay Cycle for Select1/1 -> RFC_IQ_RX_ADDR/1, [RFC_IQ_RX_ADDR_SCOPE]
  RFA Delay Cycle for Select2/1 -> RFC_IQ_RX_WEN/1, [RFC_IQ_RX_WEN_SCOPE]
  Constant17/1 -> RFC_IQ_TX_DIN/1
  RFA Delay Cycle for Select3/1 -> RFC_IQ_RX_DOUT/1, [RFC_IQ_RX_DOUT_SCOPE]
  Concat1/1 -> RFA Delay Cycle for Select3/1
  RFA Delay Cycle for Select4/1 -> RFC_IQ_TX_ADDR/1, [RFC_IQ_TX_ADDR_SCOPE]
  RFA Delay Cycle for Select5/1 -> Delay Cycle for Select/1
  IQ_RX_ADDR[1:0]/1 -> Inverter/1, Mux/2
  Inverter/1 -> Mux/3
  Mux/1 -> Mux1/1
  Inverter1/1 -> Mux2/3
  Delay Cycle for Select/1 -> Inverter1/1, Mux2/2
  Mux2/1 -> Mux3/1, [RFC_IQ_TX_SEL_SCOPE]
  [RX_WORD_ORDER] -> Mux/1
  Mux3/1 -> IQ_TX_DOUT/1, [RFC_IQ_TX_DOUT_SCOPE]
  RSSI_ADDR/1 -> RSSI_ADDR[1:0]/1, RSSI_ADDR[N:2]/1
  RFC_RSSI_ADDR/1 -> Terminator5/1
  RFC_RSSI_WEN/1 -> Terminator6/1
  RFC_RSSI_DOUT/1 -> Terminator1/1
  RFC_RSSI_ENABLE/1 -> Terminator3/1
  RFC_RSSI_RESET/1 -> Terminator4/1
  RFC_RSSI_DIN/1 -> Terminator2/1
  Constant11/1 -> RFC_RSSI_RESET/1
  Constant3/1 -> RFC_RSSI_ENABLE/1
  Constant6/1 -> RFC_RSSI_DIN/1
  Constant5/1 -> Concat8/1
  RSSI_ADDR[N:2]/1 -> Concat8/2
  Constant4/1 -> Concat8/3
  Concat8/1 -> RFA Delay Cycle for Select6/1
  RFA Delay Cycle for Select6/1 -> RFC_RSSI_ADDR/1, Gateway Out1/1
  RFA Delay Cycle for Select7/1 -> RFC_RSSI_WEN/1, Gateway Out2/1
  RFA Delay Cycle for Select8/1 -> RFC_RSSI_DOUT/1, Gateway Out3/1
  RSSI_ADDR[1:0]/1 -> Inverter2/1, Mux4/2
  Inverter2/1 -> Mux4/3
  Gateway Out1/1 -> RSSI Mem Interface/1
  Gateway Out2/1 -> RSSI Mem Interface/2
  Gateway Out3/1 -> RSSI Mem Interface/3
  Constant15/1 -> Concat3/1, Concat3/2, Concat3/3, Concat3/4
  IQ_RX_WEN/1 -> Concat3/13, Concat3/14, Concat3/15, Concat3/16, Concat2/9, Concat2/10, Concat2/11, Concat2/12, Concat11/5, Concat11/6, Concat11/7, Concat11/8, Concat10/1, Concat10/2, Concat10/3, Concat10/4
  Constant16/1 -> Concat2/1, Concat2/2, Concat2/3, Concat2/4
  Constant23/1 -> Concat2/13, Concat2/14, Concat2/15, Concat2/16
  Constant22/1 -> Concat11/3, Concat11/4, Concat11/2, Concat11/1
  Constant24/1 -> Concat11/15, Concat11/16, Concat11/14, Concat11/13
  Constant26/1 -> Concat11/11, Concat11/12, Concat11/10, Concat11/9
  Constant27/1 -> Concat10/15, Concat10/16, Concat10/14, Concat10/13
  Constant19/1 -> Concat10/11, Concat10/12, Concat10/10, Concat10/9
  Constant28/1 -> Concat10/7, Concat10/8, Concat10/6, Concat10/5
  Constant29/1 -> Concat2/7, Concat2/8, Concat2/6, Concat2/5
  Constant30/1 -> Concat3/11, Concat3/12, Concat3/10, Concat3/9
  Constant31/1 -> Concat3/7, Concat3/8, Concat3/6, Concat3/5
  Concat3/1 -> Mux1/2
  Concat2/1 -> Mux1/3
  Concat11/1 -> Mux1/4
  Concat10/1 -> Mux1/5
  [RX_WORD_ORDER] -> Mux4/1
  [TX_WORD_ORDER] -> Mux2/1
  RSSI_DIN/1 -> Concat5/4, Concat5/3, Concat5/2, Concat5/1
  Mux5/1 -> RFA Delay Cycle for Select7/1
  Concat5/1 -> RFA Delay Cycle for Select8/1
  Mux4/1 -> Mux5/1
  Constant7/1 -> Concat13/1, Concat13/2, Concat13/3, Concat13/4
  RSSI_WEN/1 -> Concat13/13, Concat13/14, Concat13/15, Concat13/16, Concat12/9, Concat12/10, Concat12/11, Concat12/12, Concat7/5, Concat7/6, Concat7/7, Concat7/8, Concat6/1, Concat6/2, Concat6/3, Concat6/4
  Constant8/1 -> Concat12/1, Concat12/2, Concat12/3, Concat12/4
  Constant34/1 -> Concat12/13, Concat12/14, Concat12/15, Concat12/16
  Constant33/1 -> Concat7/3, Concat7/4, Concat7/2, Concat7/1
  Constant35/1 -> Concat7/15, Concat7/16, Concat7/14, Concat7/13
  Constant36/1 -> Concat7/11, Concat7/12, Concat7/10, Concat7/9
  Constant37/1 -> Concat6/15, Concat6/16, Concat6/14, Concat6/13
  Constant32/1 -> Concat6/11, Concat6/12, Concat6/10, Concat6/9
  Constant38/1 -> Concat6/7, Concat6/8, Concat6/6, Concat6/5
  Constant39/1 -> Concat12/7, Concat12/8, Concat12/6, Concat12/5
  Constant40/1 -> Concat13/11, Concat13/12, Concat13/10, Concat13/9
  Constant41/1 -> Concat13/7, Concat13/8, Concat13/6, Concat13/5
  Concat13/1 -> Mux5/2
  Concat12/1 -> Mux5/3
  Concat7/1 -> Mux5/4
  Concat6/1 -> Mux5/5
  IQ_TX_DIN[95:64]/1 -> Mux3/4
  IQ_TX_DIN[127:96]/1 -> Mux3/5
